simulink subsystem "MCI"  (R2023b)
settings: Solver=VariableStepAuto  StartTime=0.0  StopTime=10.0  RelTol=1e-3
settings Model: Creator=Usuario_UMA  LastModifiedBy=Usuario_UMA

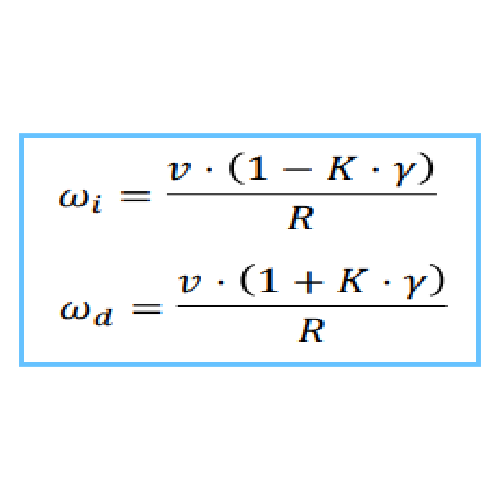
[thumbnail: Simulink's stored preview of the top-level diagram]
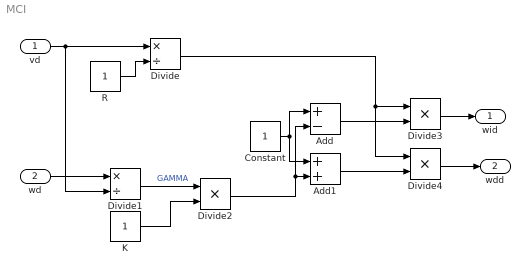
== system MCI ==
  vd : Inport
  wd : Inport  Port=2
  Add : Sum  Inputs=+-
  Add1 : Sum
  Constant : Constant
  Divide : Product  Inputs=*/
  Divide1 : Product  Inputs=*/
  Divide2 : Product  Inputs=**
  Divide3 : Product  Inputs=**
  Divide4 : Product  Inputs=**
  K : Constant
  R : Constant
  wid : Outport
  wdd : Outport  Port=2
  wires:
  vd/1 -> Divide/1, Divide1/2
  R/1 -> Divide/2
  wd/1 -> Divide1/1
  Divide1/1 -> Divide2/1  "GAMMA"
  Constant/1 -> Add1/1, Add/1
  K/1 -> Divide2/2
  Divide2/1 -> Add1/2, Add/2
  Divide/1 -> Divide3/1, Divide4/1
  Add/1 -> Divide3/2
  Add1/1 -> Divide4/2
  Divide4/1 -> wdd/1
  Divide3/1 -> wid/1
